simulink model "MotorDriveThermalTestbench"  (R2024b)
settings: Solver=daessc  StartTime=0.0  StopTime=2400  FixedStep=dt  RelTol=1e-3  AbsTol=1e-3
PreLoadFcn:
  | % Simulation parameters
  | MotorDriveThermalTestBenchParams;
model workspace (MAT data in the model file):
  V_frac_bridge = 0.0437
  V_fract_teeth = 0.9563
values from neighbouring files (symbols this model uses):
  CaseParams = struct()    [InverterThermalParams.m]
  HeatsinkParams = struct()    [InverterThermalParams.m]
undefined symbols (not defined in the file or in its folder): electricDrive, H_AH, H_AL, H_BH, H_BL, H_CH, H_CL, PipeParams, vehicleThermal
libraries: fl_lib x171, ee_lib x31, nesl_utility x28, nesl_utility_internal x12, sdl_lib x6, SimscapeFluids_lib x3, autolibshared x1
(part 3 of 4)

== system MotorDriveThermalTestbench/Inverter/AbstractInverter /Inverter Power Module Thermal/HeatSink ==
  Flow Rate Sensor : fl_lib/Thermal Liquid/Sensors/Flow Rate Sensor (TL)  mass_flow_measure=false  volumetric_flow_measure=true  energy_flow_measure=false
      settings: InternalSimscapePortConfiguration="{\"Bottom\":[],\"Left\":[{\"id\":\"A\",\"label\":\"A\",\"type\":\"foundation.thermal_liquid.thermal_liquid\"}],\"Right\":[{\"id\":\"B\",\"label\":\"B\",\"type\":\"foundation.thermal_liquid.thermal_liquid\"},{\"id\":\"V\",\"label\":\"V\",\"type\":\"output\"}],\"Top\":[]}"
  HS Eq Pipe : fl_lib/Thermal Liquid/Elements/Pipe (TL)  length=1.1*HeatsinkParams.ChennelLength m  area=HeatsinkParams.EqPipeDia^2*pi/4 m^2  Dh=HeatsinkParams.EqPipeDia m  length_add=HeatsinkParams.EqLengthRough m  roughness=HeatsinkParams.EqPipeRoughness m  Re_lam=2000  Re_tur=4000  shape_factor=64  Nu_lam=3000  dynamic_compressibility=simscape.enum.onoff.off  inertia=simscape.enum.onoff.off  p0=0.101325 MPa  T0=Tamb degC  mdot0=0 kg/s
  Heatsink : ee_lib/Passive/Thermal/Heatsink  parameterization=ee.enum.passive.thermal.heatsinkParam.rectangularFin  convection=ee.enum.passive.thermal.heatsinkConvection.specifyFlowSpeed  T_vec_Q=[10, 30, 50, 70, 90] K  v_vec_Q=[0, 1, 2, 3] m/s  Q_TLU1=[6.1, 23.6, 44.5, 67.5, 92.3] W  Q_TLU2=[6.1, 18.8, 22.8, 25.7; 23.6, 61.1, 73, 81.5; 44.5, 106.4, 125.9, 140.1; 67.5, 153.5, 180.7, 200.3; 92.3, 202.1, 236.9, 262] W  T_vec_h=[10, 30, 50, 70, 90] K  v_vec_h=[0, 1, 2, 3] m/s  h_TLU1=[5.4, 7.02, 7.98, 8.68, 9.26] W/(K*m^2)  h_TLU2=[5.4, 17.86, 22.17, 25.41; 7.02, 19.49, 23.8, 27.03; 7.97, 20.44, 24.75, 27.99; 8.68, 21.15, 25.46, 28.69; 9.26, 21.73, 26.04, 29.27] W/(K*m^2)  h_vec=[5, 10, 15, 20, 25, 30] W/(K*m^2)  eff_TLU=[96.97, 94.16, 91.53, 89.08, 86.78, 84.62]  height=electricDrive.HeatsinkParams.Height m  thick=electricDrive.HeatsinkParams.Thick m  depth=electricDrive.HeatsinkParams.Depth m  gap=electricDrive.HeatsinkParams.Gap m  num_fins=electricDrive.HeatsinkParams.NumFins  k_fin=386 W/(K*m)  A_total=0.1171 m^2  nu=2.62e-6 m^2/s  alpha=6.55e-8 m^2/s  k_fluid=0.55 W/(K*m)  beta=5.82e-4 1/K  mass=electricDrive.HeatsinkParams.Mass kg  sp_heat=437 J/(K*kg)  T_hs_specify=on  T_hs_priority=High  T_hs=electricDrive.PMparams.TinitCase K  T_hs_nominal_specify=off  T_hs_nominal_value=1  T_hs_nominal_unit=K  Q_A_specify=off  Q_A_priority=None  Q_A=0 W  Q_A_nominal_specify=on  Q_A_nominal_value=1  Q_A_nominal_unit=W  Q_C_specify=off  Q_C_priority=None  Q_C=0 W  Q_C_nominal_specify=on  Q_C_nominal_value=1  Q_C_nominal_unit=W
      settings: InternalSimscapePortConfiguration="{\"Bottom\":[{\"id\":\"C\",\"label\":\"C\",\"type\":\"foundation.thermal.thermal\"}],\"Left\":[{\"id\":\"v\",\"label\":\"v\",\"type\":\"input\"}],\"Right\":[],\"Top\":[{\"id\":\"A\",\"label\":\"A\",\"type\":\"foundation.thermal.thermal\"}]}"
  PS Constant1 : fl_lib/Physical Signals/Sources/PS Constant  constant=PipeParams.Diameter^2*pi/4 m^2
  PS Divide : fl_lib/Physical Signals/Functions/PS Divide
  PS-Simulink Converter : nesl_utility/PS-Simulink Converter  PhysicalDomain=network_engine_domain  SubClassName=ps_output  LeftPortType=input  RightPortType=output  PseudoPeriodic=off  Frequencies=[]  VectorFormat=inherit  Unit=inherit  AffineConversion=off
  Pressure & Temperature Sensor (TL) : fl_lib/Thermal Liquid/Sensors/Pressure & Temperature Sensor (TL)  reference=foundation.enum.MeasurementReference.difference  pressure=true  pressure_spec=foundation.enum.PressureMeasementSpec.Absolute  temperature=true
      settings: InternalSimscapePortConfiguration="{\"Bottom\":[{\"id\":\"T\",\"label\":\"T\",\"type\":\"output\"}],\"Left\":[{\"id\":\"A\",\"label\":\"A\",\"type\":\"foundation.thermal_liquid.thermal_liquid\"}],\"Right\":[{\"id\":\"B\",\"label\":\"B\",\"type\":\"foundation.thermal_liquid.thermal_liquid\"},{\"id\":\"P\",\"label\":\"P\",\"type\":\"output\"}],\"Top\":[]}"
  Scope : Scope
  Hinv : PMIOPort  Side=Left
  coolantIn : PMIOPort  Port=2  Side=Left
  coolantOut : PMIOPort  Port=3  Side=Right
  wires:
  PS-Simulink Converter/1 -> Scope/1
  connections:
  PS Divide/RConn1 -- Heatsink/LConn1
  HS Eq Pipe/LConn1 -- Pressure & Temperature Sensor (TL)/RConn1 -- coolantOut/RConn1
  HS Eq Pipe/RConn1 -- Pressure & Temperature Sensor (TL)/LConn1 -- Flow Rate Sensor/RConn1
  coolantIn/RConn1 -- Flow Rate Sensor/LConn1
  PS Constant1/RConn1 -- PS Divide/LConn2
  Flow Rate Sensor/RConn2 -- PS Divide/LConn1
  HS Eq Pipe/LConn2 -- Heatsink/LConn2
  Hinv/RConn1 -- Heatsink/RConn1
  PS-Simulink Converter/LConn1 -- Pressure & Temperature Sensor (TL)/RConn2

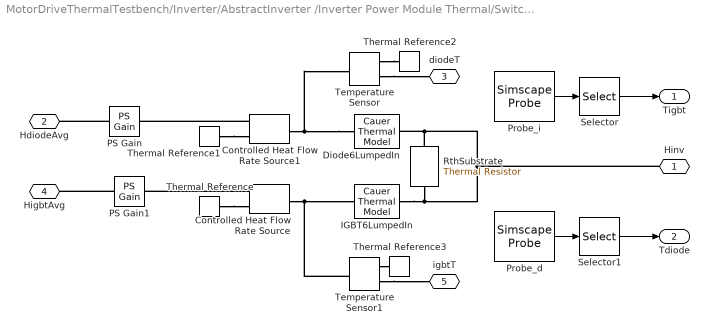
== system MotorDriveThermalTestbench/Inverter/AbstractInverter /Inverter Power Module Thermal/Switches(Averaged IGBT Diode) ==
  Controlled Heat Flow Rate Source : fl_lib/Thermal/Thermal Sources/Controlled Heat Flow Rate Source
  Controlled Heat Flow Rate Source1 : fl_lib/Thermal/Thermal Sources/Controlled Heat Flow Rate Source
  Diode6LumpedIn : ee_lib/Passive/Thermal/Cauer Thermal Model  parameterize_foster=true  resistance_data=1e-3 * [2.6468, 3.8701, 1.2007, .8824] K/W  tau_data=[.0086, .054, .3624, 1.651] s  resistance_data_foster=electricDrive.PMparams.RthDiode K/W  tau_data_foster=electricDrive.PMparams.tauthDiode s  Tvec_specify=on  Tvec_priority=High  Tvec=electricDrive.PMparams.TinitDiode deltaK  Tvec_nominal_specify=off  Tvec_nominal_value=1  Tvec_nominal_unit=K  Q_A_specify=off  Q_A_priority=None  Q_A=0 W  Q_A_nominal_specify=off  Q_A_nominal_value=1  Q_A_nominal_unit=W  Q_B_specify=off  Q_B_priority=None  Q_B=0 W  Q_B_nominal_specify=off  Q_B_nominal_value=1  Q_B_nominal_unit=W
      settings: InternalSimscapePortConfiguration="{\"Bottom\":[],\"Left\":[{\"id\":\"A\",\"label\":\"A\",\"type\":\"foundation.thermal.thermal\"}],\"Right\":[{\"id\":\"B\",\"label\":\"B\",\"type\":\"foundation.thermal.thermal\"}],\"Top\":[]}"
  IGBT6LumpedIn : ee_lib/Passive/Thermal/Cauer Thermal Model  parameterize_foster=true  resistance_data=1e-3 * [2.6468, 3.8701, 1.2007, .8824] K/W  tau_data=[.0086, .054, .3624, 1.651] s  resistance_data_foster=electricDrive.PMparams.RthIGBT K/W  tau_data_foster=electricDrive.PMparams.tauthIGBT s  Tvec_specify=on  Tvec_priority=High  Tvec=electricDrive.PMparams.TinitIGBT deltaK  Tvec_nominal_specify=off  Tvec_nominal_value=1  Tvec_nominal_unit=K  Q_A_specify=off  Q_A_priority=None  Q_A=0 W  Q_A_nominal_specify=off  Q_A_nominal_value=1  Q_A_nominal_unit=W  Q_B_specify=off  Q_B_priority=None  Q_B=0 W  Q_B_nominal_specify=off  Q_B_nominal_value=1  Q_B_nominal_unit=W
      settings: InternalSimscapePortConfiguration="{\"Bottom\":[],\"Left\":[{\"id\":\"A\",\"label\":\"A\",\"type\":\"foundation.thermal.thermal\"}],\"Right\":[{\"id\":\"B\",\"label\":\"B\",\"type\":\"foundation.thermal.thermal\"}],\"Top\":[]}"
  PS Gain : fl_lib/Physical Signals/Functions/PS Gain  gain=6 J/s
  PS Gain1 : fl_lib/Physical Signals/Functions/PS Gain  gain=6 J/s
  Probe_d : SimscapeProbe  BoundBlock=3849  Variables={Tvec}
  Probe_i : SimscapeProbe  BoundBlock=3850  Variables={Tvec}
  RthSubstrate : ee_lib/Passive/Thermal/Thermal Resistor  R=1e-2 K/W  T_specify=off  T_priority=None  T=0 K  T_nominal_specify=off  T_nominal_value=1  T_nominal_unit=K  Q_specify=off  Q_priority=None  Q=0 W  Q_nominal_specify=off  Q_nominal_value=1  Q_nominal_unit=W
      settings: InternalSimscapePortConfiguration="{\"Bottom\":[],\"Left\":[{\"id\":\"A\",\"label\":\"A\",\"type\":\"foundation.thermal.thermal\"}],\"Right\":[{\"id\":\"B\",\"label\":\"B\",\"type\":\"foundation.thermal.thermal\"}],\"Top\":[]}"
  Selector : Selector  InputPortWidth=4  IndexOptions=Index vector (dialog)  Indices=[1]  OutputSizes=1
  Selector1 : Selector  InputPortWidth=4  IndexOptions=Index vector (dialog)  Indices=[1]  OutputSizes=1
  Temperature Sensor : fl_lib/Thermal/Thermal Sensors/Temperature Sensor  temperature_measure=foundation.enum.MeasurementReference.difference
  Temperature Sensor1 : fl_lib/Thermal/Thermal Sensors/Temperature Sensor  temperature_measure=foundation.enum.MeasurementReference.difference
  Thermal Reference{,1..3} (4 alike) : fl_lib/Thermal/Thermal Elements/Thermal Reference
  Hinv : PMIOPort  Side=Left
  HdiodeAvg : PMIOPort  Port=2  Side=Right
  diodeT : PMIOPort  Port=3  Side=Right
  HigbtAvg : PMIOPort  Port=4  Side=Right
  igbtT : PMIOPort  Port=5  Side=Right
  Tigbt : Outport
  Tdiode : Outport  Port=2
  wires:
  Probe_d/1 -> Selector1/1
  Probe_i/1 -> Selector/1
  Selector/1 -> Tigbt/1
  Selector1/1 -> Tdiode/1
  connections:
  Thermal Reference/LConn1 -- Controlled Heat Flow Rate Source/RConn2
  Diode6LumpedIn/LConn1 -- Temperature Sensor/LConn1 -- Controlled Heat Flow Rate Source1/LConn1
  Controlled Heat Flow Rate Source1/RConn1 -- PS Gain/RConn1
  RthSubstrate/LConn1 -- IGBT6LumpedIn/RConn1 -- Hinv/RConn1 -- RthSubstrate/RConn1 -- Diode6LumpedIn/RConn1
  Thermal Reference1/LConn1 -- Controlled Heat Flow Rate Source1/RConn2
  Controlled Heat Flow Rate Source/RConn1 -- PS Gain1/RConn1
  Temperature Sensor/RConn2 -- diodeT/RConn1
  Temperature Sensor/RConn1 -- Thermal Reference2/LConn1
  Temperature Sensor1/RConn1 -- Thermal Reference3/LConn1
  Temperature Sensor1/RConn2 -- igbtT/RConn1
  Temperature Sensor1/LConn1 -- Controlled Heat Flow Rate Source/LConn1 -- IGBT6LumpedIn/LConn1
  PS Gain/LConn1 -- HdiodeAvg/RConn1
  PS Gain1/LConn1 -- HigbtAvg/RConn1

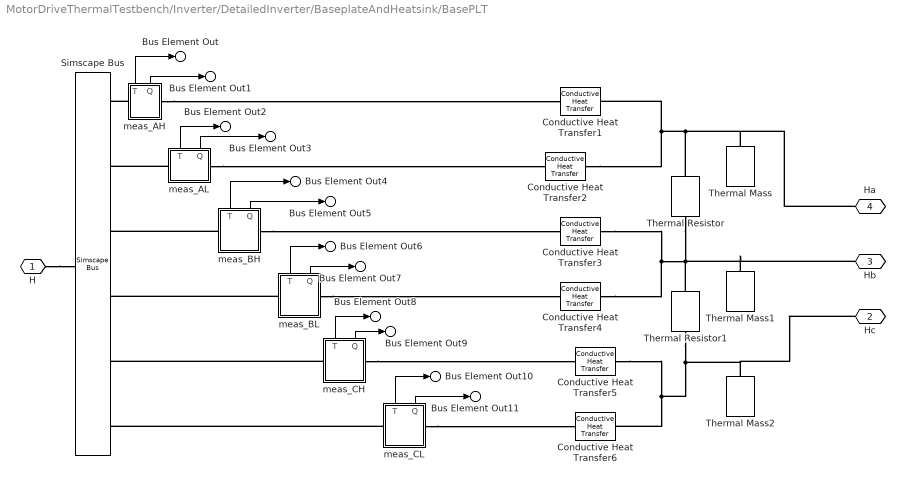
== system MotorDriveThermalTestbench/Inverter/DetailedInverter/BaseplateAndHeatsink/BasePLT ==
  Conductive Heat Transfer{1..6} (6 alike) : fl_lib/Thermal/Thermal Elements/Conductive Heat Transfer  thermal_type=foundation.enum.ConstantVariableTabulated.Constant  wall_geometry=foundation.enum.ConductionWallGeometry.Planar  area=CaseParams.Area m^2  thickness=CaseParams.Thickness m  d_in=0.05 m  d_out=0.1 m  L=1 m  th_cond_min=10 W/(K*m)  th_cond=CaseParams.ThermalConductivity W/(K*m)  th_cond_TLU=[413, 401, 392, 383, 371, 357, 342] W/(K*m)  temp_TLU=[200, 273, 400, 600, 800, 1000, 1200] K  T_specify=off  T_priority=None  T=0 K  T_nominal_specify=off  T_nominal_value=1  T_nominal_unit=K  Q_specify=off  Q_priority=None  Q=0 W  Q_nominal_specify=off  Q_nominal_value=1  Q_nominal_unit=W
  Simscape Bus : SimscapeBus  HierarchyStrings=H_AH;H_AL;H_BH;H_BL;H_CH;H_CL
  Thermal Mass : fl_lib/Thermal/Thermal Elements/Thermal Mass  mass_type=foundation.enum.constant_variable.constant  mass=CaseParams.Mass/3 kg  sp_heat=CaseParams.SpHeat J/(K*kg)  mass_min=1e-6 kg  num_ports=foundation.enum.numPorts2.one  m_specify=off  m_priority=High  m=1 kg  m_nominal_specify=off  m_nominal_value=1  m_nominal_unit=kg  T_specify=on  T_priority=High  T=electricDrive.PMparams.TinitCase K  T_nominal_specify=off  T_nominal_value=1  T_nominal_unit=K  Q_specify=off  Q_priority=None  Q=0 W  Q_nominal_specify=off  Q_nominal_value=1  Q_nominal_unit=W
  Thermal Mass1 : fl_lib/Thermal/Thermal Elements/Thermal Mass  mass_type=foundation.enum.constant_variable.constant  mass=CaseParams.Mass/3 kg  sp_heat=CaseParams.SpHeat J/(K*kg)  mass_min=1e-6 kg  num_ports=foundation.enum.numPorts2.one  m_specify=off  m_priority=High  m=1 kg  m_nominal_specify=off  m_nominal_value=1  m_nominal_unit=kg  T_specify=on  T_priority=High  T=electricDrive.PMparams.TinitCase K  T_nominal_specify=off  T_nominal_value=1  T_nominal_unit=K  Q_specify=off  Q_priority=None  Q=0 W  Q_nominal_specify=off  Q_nominal_value=1  Q_nominal_unit=W
  Thermal Mass2 : fl_lib/Thermal/Thermal Elements/Thermal Mass  mass_type=foundation.enum.constant_variable.constant  mass=CaseParams.Mass/3 kg  sp_heat=CaseParams.SpHeat J/(K*kg)  mass_min=1e-6 kg  num_ports=foundation.enum.numPorts2.one  m_specify=off  m_priority=High  m=1 kg  m_nominal_specify=off  m_nominal_value=1  m_nominal_unit=kg  T_specify=on  T_priority=High  T=electricDrive.PMparams.TinitCase K  T_nominal_specify=off  T_nominal_value=1  T_nominal_unit=K  Q_specify=off  Q_priority=None  Q=0 W  Q_nominal_specify=off  Q_nominal_value=1  Q_nominal_unit=W
  Thermal Resistor : ee_lib/Passive/Thermal/Thermal Resistor  R=1e-1 K/W  T_specify=off  T_priority=None  T=0 K  T_nominal_specify=off  T_nominal_value=1  T_nominal_unit=K  Q_specify=off  Q_priority=None  Q=0 W  Q_nominal_specify=off  Q_nominal_value=1  Q_nominal_unit=W
      settings: InternalSimscapePortConfiguration="{\"Bottom\":[],\"Left\":[{\"id\":\"A\",\"label\":\"A\",\"type\":\"foundation.thermal.thermal\"}],\"Right\":[{\"id\":\"B\",\"label\":\"B\",\"type\":\"foundation.thermal.thermal\"}],\"Top\":[]}"
  Thermal Resistor1 : ee_lib/Passive/Thermal/Thermal Resistor  R=1e-1 K/W  T_specify=off  T_priority=None  T=0 K  T_nominal_specify=off  T_nominal_value=1  T_nominal_unit=K  Q_specify=off  Q_priority=None  Q=0 W  Q_nominal_specify=off  Q_nominal_value=1  Q_nominal_unit=W
      settings: InternalSimscapePortConfiguration="{\"Bottom\":[],\"Left\":[{\"id\":\"A\",\"label\":\"A\",\"type\":\"foundation.thermal.thermal\"}],\"Right\":[{\"id\":\"B\",\"label\":\"B\",\"type\":\"foundation.thermal.thermal\"}],\"Top\":[]}"
  meas_AH : Subsystem
      settings: PortSchema="{\"entries\":[{\"content\":{\"sides\":[{\"content\":{\"connectorIds\":[\"LConn1\"]},\"type\":\"ConnectorPlacement.EquallySpacedRectSide\",\"uuid\":\"1fc63631-1283-41fa-989f-998ad8911336\"},{\"content\":{\"connectorIds\":[\"RConn1\"],\"side\":\"RIGHT\"},\"type\":\"ConnectorPlacement.EquallySpacedRectSide\",\"uuid\":\"60331112-9c9a-4116-97c9-fe3ae6fff227\"},{\"content\":{\"connectorIds\":[\"Out1\",\"Out2\"],\"side\":\"TOP\"},\"type\":\"ConnectorPlacement.EquallySpacedRectSide\",\"uuid\":\"96faf64b-4185-4f1f-9fc5-9c6afe90db96\"}]},\"type\":\"ConnectorPlacement.EquallySpacedConnector\",\"uuid\":\"7d6ee35a-d18e-4643-9192-adf0d71fa59d\"}],\"packageUris\":[\"http://schema.mathworks.com/mf0/Connector/R2020b\"],\"version\":\"1.0\"}"
  meas_AL : Subsystem
      settings: PortSchema="{\"entries\":[{\"content\":{\"sides\":[{\"content\":{\"connectorIds\":[\"LConn1\"]},\"type\":\"ConnectorPlacement.EquallySpacedRectSide\",\"uuid\":\"1fc63631-1283-41fa-989f-998ad8911336\"},{\"content\":{\"connectorIds\":[\"RConn1\"],\"side\":\"RIGHT\"},\"type\":\"ConnectorPlacement.EquallySpacedRectSide\",\"uuid\":\"60331112-9c9a-4116-97c9-fe3ae6fff227\"},{\"content\":{\"connectorIds\":[\"Out1\",\"Out2\"],\"side\":\"TOP\"},\"type\":\"ConnectorPlacement.EquallySpacedRectSide\",\"uuid\":\"96faf64b-4185-4f1f-9fc5-9c6afe90db96\"}]},\"type\":\"ConnectorPlacement.EquallySpacedConnector\",\"uuid\":\"7d6ee35a-d18e-4643-9192-adf0d71fa59d\"}],\"packageUris\":[\"http://schema.mathworks.com/mf0/Connector/R2020b\"],\"version\":\"1.0\"}"
  meas_BH : Subsystem
      settings: PortSchema="{\"entries\":[{\"content\":{\"sides\":[{\"content\":{\"connectorIds\":[\"LConn1\"]},\"type\":\"ConnectorPlacement.EquallySpacedRectSide\",\"uuid\":\"1fc63631-1283-41fa-989f-998ad8911336\"},{\"content\":{\"connectorIds\":[\"RConn1\"],\"side\":\"RIGHT\"},\"type\":\"ConnectorPlacement.EquallySpacedRectSide\",\"uuid\":\"60331112-9c9a-4116-97c9-fe3ae6fff227\"},{\"content\":{\"connectorIds\":[\"Out1\",\"Out2\"],\"side\":\"TOP\"},\"type\":\"ConnectorPlacement.EquallySpacedRectSide\",\"uuid\":\"96faf64b-4185-4f1f-9fc5-9c6afe90db96\"}]},\"type\":\"ConnectorPlacement.EquallySpacedConnector\",\"uuid\":\"7d6ee35a-d18e-4643-9192-adf0d71fa59d\"}],\"packageUris\":[\"http://schema.mathworks.com/mf0/Connector/R2020b\"],\"version\":\"1.0\"}"
  meas_BL : Subsystem
      settings: PortSchema="{\"entries\":[{\"content\":{\"sides\":[{\"content\":{\"connectorIds\":[\"LConn1\"]},\"type\":\"ConnectorPlacement.EquallySpacedRectSide\",\"uuid\":\"1fc63631-1283-41fa-989f-998ad8911336\"},{\"content\":{\"connectorIds\":[\"RConn1\"],\"side\":\"RIGHT\"},\"type\":\"ConnectorPlacement.EquallySpacedRectSide\",\"uuid\":\"60331112-9c9a-4116-97c9-fe3ae6fff227\"},{\"content\":{\"connectorIds\":[\"Out1\",\"Out2\"],\"side\":\"TOP\"},\"type\":\"ConnectorPlacement.EquallySpacedRectSide\",\"uuid\":\"96faf64b-4185-4f1f-9fc5-9c6afe90db96\"}]},\"type\":\"ConnectorPlacement.EquallySpacedConnector\",\"uuid\":\"7d6ee35a-d18e-4643-9192-adf0d71fa59d\"}],\"packageUris\":[\"http://schema.mathworks.com/mf0/Connector/R2020b\"],\"version\":\"1.0\"}"
  meas_CH : Subsystem
      settings: PortSchema="{\"entries\":[{\"content\":{\"sides\":[{\"content\":{\"connectorIds\":[\"LConn1\"]},\"type\":\"ConnectorPlacement.EquallySpacedRectSide\",\"uuid\":\"1fc63631-1283-41fa-989f-998ad8911336\"},{\"content\":{\"connectorIds\":[\"RConn1\"],\"side\":\"RIGHT\"},\"type\":\"ConnectorPlacement.EquallySpacedRectSide\",\"uuid\":\"60331112-9c9a-4116-97c9-fe3ae6fff227\"},{\"content\":{\"connectorIds\":[\"Out1\",\"Out2\"],\"side\":\"TOP\"},\"type\":\"ConnectorPlacement.EquallySpacedRectSide\",\"uuid\":\"96faf64b-4185-4f1f-9fc5-9c6afe90db96\"}]},\"type\":\"ConnectorPlacement.EquallySpacedConnector\",\"uuid\":\"7d6ee35a-d18e-4643-9192-adf0d71fa59d\"}],\"packageUris\":[\"http://schema.mathworks.com/mf0/Connector/R2020b\"],\"version\":\"1.0\"}"
  meas_CL : Subsystem
      settings: PortSchema="{\"entries\":[{\"content\":{\"sides\":[{\"content\":{\"connectorIds\":[\"LConn1\"]},\"type\":\"ConnectorPlacement.EquallySpacedRectSide\",\"uuid\":\"1fc63631-1283-41fa-989f-998ad8911336\"},{\"content\":{\"connectorIds\":[\"RConn1\"],\"side\":\"RIGHT\"},\"type\":\"ConnectorPlacement.EquallySpacedRectSide\",\"uuid\":\"60331112-9c9a-4116-97c9-fe3ae6fff227\"},{\"content\":{\"connectorIds\":[\"Out1\",\"Out2\"],\"side\":\"TOP\"},\"type\":\"ConnectorPlacement.EquallySpacedRectSide\",\"uuid\":\"96faf64b-4185-4f1f-9fc5-9c6afe90db96\"}]},\"type\":\"ConnectorPlacement.EquallySpacedConnector\",\"uuid\":\"7d6ee35a-d18e-4643-9192-adf0d71fa59d\"}],\"packageUris\":[\"http://schema.mathworks.com/mf0/Connector/R2020b\"],\"version\":\"1.0\"}"
  H : PMIOPort  Tag=PMCPort  Side=Left
  Hc : PMIOPort  Port=2  Side=Right
  Hb : PMIOPort  Port=3  Side=Right
  Ha : PMIOPort  Port=4  Side=Right
  Bus Element Out : Outport  PortName=Tmeas  Element=T_AH
  Bus Element Out1 : Outport  PortName=Tmeas  Element=Q_AH
  Bus Element Out2 : Outport  PortName=Tmeas  Element=T_AL
  Bus Element Out3 : Outport  PortName=Tmeas  Element=Q_AL
  Bus Element Out4 : Outport  PortName=Tmeas  Element=T_BH
  Bus Element Out5 : Outport  PortName=Tmeas  Element=Q_BH
  Bus Element Out6 : Outport  PortName=Tmeas  Element=T_BL
  Bus Element Out7 : Outport  PortName=Tmeas  Element=Q_BL
  Bus Element Out8 : Outport  PortName=Tmeas  Element=T_CH
  Bus Element Out9 : Outport  PortName=Tmeas  Element=Q_CH
  Bus Element Out10 : Outport  PortName=Tmeas  Element=T_CL
  Bus Element Out11 : Outport  PortName=Tmeas  Element=Q_CL
  wires:
  meas_AH/1(T) -> Bus Element Out/1
  meas_AH/2(Q) -> Bus Element Out1/1
  meas_AL/1(T) -> Bus Element Out2/1
  meas_AL/2(Q) -> Bus Element Out3/1
  meas_BH/1(T) -> Bus Element Out4/1
  meas_BH/2(Q) -> Bus Element Out5/1
  meas_BL/2(Q) -> Bus Element Out7/1
  meas_BL/1(T) -> Bus Element Out6/1
  meas_CH/2(Q) -> Bus Element Out9/1
  meas_CH/1(T) -> Bus Element Out8/1
  meas_CL/2(Q) -> Bus Element Out11/1
  meas_CL/1(T) -> Bus Element Out10/1
  connections:
  H/RConn1 -- Simscape Bus/RConn1
  Conductive Heat Transfer2/RConn1 -- Thermal Mass/LConn1 -- Ha/RConn1 -- Thermal Resistor/LConn1 -- Conductive Heat Transfer1/RConn1
  meas_AH/RConn1 -- Conductive Heat Transfer1/LConn1
  meas_AH/LConn1 -- Simscape Bus/LConn1
  meas_AL/LConn1 -- Simscape Bus/LConn2
  meas_AL/RConn1 -- Conductive Heat Transfer2/LConn1
  meas_BH/LConn1 -- Simscape Bus/LConn3
  meas_BH/RConn1 -- Conductive Heat Transfer3/LConn1
  meas_BL/RConn1 -- Conductive Heat Transfer4/LConn1
  meas_BL/LConn1 -- Simscape Bus/LConn4
  meas_CH/LConn1 -- Simscape Bus/LConn5
  meas_CH/RConn1 -- Conductive Heat Transfer5/LConn1
  meas_CL/LConn1 -- Simscape Bus/LConn6
  meas_CL/RConn1 -- Conductive Heat Transfer6/LConn1
  Conductive Heat Transfer3/RConn1 -- Conductive Heat Transfer4/RConn1 -- Thermal Resistor/RConn1 -- Thermal Mass1/LConn1 -- Hb/RConn1 -- Thermal Resistor1/LConn1
  Conductive Heat Transfer5/RConn1 -- Thermal Resistor1/RConn1 -- Hc/RConn1 -- Thermal Mass2/LConn1 -- Conductive Heat Transfer6/RConn1

== system MotorDriveThermalTestbench/Inverter/DetailedInverter/BaseplateAndHeatsink/HeatSink ==
  Flow Rate Sensor : fl_lib/Thermal Liquid/Sensors/Flow Rate Sensor (TL)  mass_flow_measure=false  volumetric_flow_measure=true  energy_flow_measure=false
      settings: InternalSimscapePortConfiguration="{\"Bottom\":[],\"Left\":[{\"id\":\"A\",\"label\":\"A\",\"type\":\"foundation.thermal_liquid.thermal_liquid\"}],\"Right\":[{\"id\":\"B\",\"label\":\"B\",\"type\":\"foundation.thermal_liquid.thermal_liquid\"},{\"id\":\"V\",\"label\":\"V\",\"type\":\"output\"}],\"Top\":[]}"
  HeatConduction : Subsystem
  HeatConvection : Subsystem
  PS Divide : fl_lib/Physical Signals/Functions/PS Divide
  PipeArea : fl_lib/Physical Signals/Sources/PS Constant  constant=PipeParams.Diameter^2*pi/4 m^2
  I : PMIOPort  Side=Left
  " Ha" : PMIOPort  Port=2  Side=Left
  Hb : PMIOPort  Port=3  Side=Left
  Hc : PMIOPort  Port=4  Side=Left
  O : PMIOPort  Port=5  Side=Right
  connections:
  HeatConduction/RConn3 -- HeatConvection/LConn4
  HeatConduction/RConn2 -- HeatConvection/LConn3
  Hc/RConn1 -- HeatConduction/LConn4
  Hb/RConn1 -- HeatConduction/LConn3
  HeatConduction/RConn1 -- HeatConvection/LConn2
  O/RConn1 -- HeatConvection/RConn1
  " Ha"/RConn1 -- HeatConduction/LConn2
  PS Divide/RConn1 -- HeatConduction/LConn1
  I/RConn1 -- Flow Rate Sensor/LConn1
  PipeArea/RConn1 -- PS Divide/LConn2
  Flow Rate Sensor/RConn2 -- PS Divide/LConn1
  Flow Rate Sensor/RConn1 -- HeatConvection/LConn1

== system MotorDriveThermalTestbench/Inverter/DetailedInverter/PowerLoss/DiodeLoss ==
  mtq : Inport
  mspd : Inport  Port=2
  temp : Inport  Port=3
  3PhaseDiodeLoss : Subsystem
  DiodeLossTbl : Subsystem
  DutyCycle : Subsystem
  LossDutyCycle : Constant  Value=0.5
  VariablePulse : Subsystem
  Hloss : Outport
  wires:
  3PhaseDiodeLoss/1(Out1) -> Hloss/1
  DutyCycle/4(timeperiod) -> VariablePulse/2(timeperiod)
  DiodeLossTbl/1(Ha) -> 3PhaseDiodeLoss/5(Ha)
  mtq/1 -> DiodeLossTbl/2(mtq)
  temp/1 -> DiodeLossTbl/3(temp)
  DiodeLossTbl/2(Hb) -> 3PhaseDiodeLoss/6(Hb)
  DiodeLossTbl/3(Hc) -> 3PhaseDiodeLoss/7(Hc)
  DutyCycle/5(MotOmega) -> DiodeLossTbl/1(momega)
  LossDutyCycle/1 -> VariablePulse/1(ds)
  DutyCycle/3(d3) -> 3PhaseDiodeLoss/3(d3)
  DutyCycle/2(d2) -> 3PhaseDiodeLoss/2(d2)
  mspd/1 -> DutyCycle/1(motRPM)
  VariablePulse/1(pulse) -> 3PhaseDiodeLoss/4(pls)
  DutyCycle/1(d1) -> 3PhaseDiodeLoss/1(d1)

== system MotorDriveThermalTestbench/Inverter/DetailedInverter/PowerLoss/IGBTloss ==
  mspd : Inport
  mtq : Inport  Port=2
  temp : Inport  Port=3
  3PhaseIGBTLoss : Subsystem
  DutyCycle : Subsystem
  IGBTLossTbl : Subsystem
  LossDutyCycle : Constant  Value=0.5
  VariablePulse : Subsystem
  loss : Outport
  wires:
  mspd/1 -> DutyCycle/1(motRPM)
  VariablePulse/1(pulse) -> 3PhaseIGBTLoss/4(pls)
  DutyCycle/4(timeperiod) -> VariablePulse/2(timeperiod)
  LossDutyCycle/1 -> VariablePulse/1(ds)
  IGBTLossTbl/3(Hc) -> 3PhaseIGBTLoss/7(Hc)
  IGBTLossTbl/2(Hb) -> 3PhaseIGBTLoss/6(Hb)
  temp/1 -> IGBTLossTbl/3(temp)
  DutyCycle/5(MotOmega) -> IGBTLossTbl/1(momega)
  IGBTLossTbl/1(Ha) -> 3PhaseIGBTLoss/5(Ha)
  3PhaseIGBTLoss/1(Out1) -> loss/1
  mtq/1 -> IGBTLossTbl/2(mtq)
  DutyCycle/2(d2) -> 3PhaseIGBTLoss/2(d2)
  DutyCycle/3(d3) -> 3PhaseIGBTLoss/3(d3)
  DutyCycle/1(d1) -> 3PhaseIGBTLoss/1(d1)

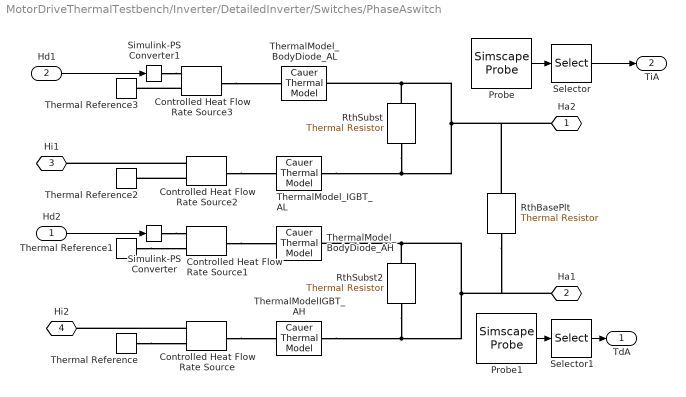
== system MotorDriveThermalTestbench/Inverter/DetailedInverter/Switches/PhaseAswitch ==
  Hd2 : Inport
  Hd1 : Inport  Port=2
  Controlled Heat Flow Rate Source{,1..3} (4 alike) : fl_lib/Thermal/Thermal Sources/Controlled Heat Flow Rate Source
  Probe : SimscapeProbe  BoundBlock=3669  Variables={Tvec}
  Probe1 : SimscapeProbe  BoundBlock=3662  Variables={Tvec}
  RthBasePlt : ee_lib/Passive/Thermal/Thermal Resistor  R=1.04 K/W  T_specify=off  T_priority=None  T=0 K  T_nominal_specify=off  T_nominal_value=1  T_nominal_unit=K  Q_specify=off  Q_priority=None  Q=0 W  Q_nominal_specify=off  Q_nominal_value=1  Q_nominal_unit=W
      settings: InternalSimscapePortConfiguration="{\"Bottom\":[],\"Left\":[{\"id\":\"A\",\"label\":\"A\",\"type\":\"foundation.thermal.thermal\"}],\"Right\":[{\"id\":\"B\",\"label\":\"B\",\"type\":\"foundation.thermal.thermal\"}],\"Top\":[]}"
  RthSubst : ee_lib/Passive/Thermal/Thermal Resistor  R=0.26 K/W  T_specify=off  T_priority=None  T=0 K  T_nominal_specify=off  T_nominal_value=1  T_nominal_unit=K  Q_specify=off  Q_priority=None  Q=0 W  Q_nominal_specify=off  Q_nominal_value=1  Q_nominal_unit=W
      settings: InternalSimscapePortConfiguration="{\"Bottom\":[],\"Left\":[{\"id\":\"A\",\"label\":\"A\",\"type\":\"foundation.thermal.thermal\"}],\"Right\":[{\"id\":\"B\",\"label\":\"B\",\"type\":\"foundation.thermal.thermal\"}],\"Top\":[]}"
  RthSubst2 : ee_lib/Passive/Thermal/Thermal Resistor  R=0.26 K/W  T_specify=off  T_priority=None  T=0 K  T_nominal_specify=off  T_nominal_value=1  T_nominal_unit=K  Q_specify=off  Q_priority=None  Q=0 W  Q_nominal_specify=off  Q_nominal_value=1  Q_nominal_unit=W
      settings: InternalSimscapePortConfiguration="{\"Bottom\":[],\"Left\":[{\"id\":\"A\",\"label\":\"A\",\"type\":\"foundation.thermal.thermal\"}],\"Right\":[{\"id\":\"B\",\"label\":\"B\",\"type\":\"foundation.thermal.thermal\"}],\"Top\":[]}"
  Selector : Selector  InputPortWidth=4  IndexOptions=Index vector (dialog)  Indices=[1]  OutputSizes=1
  Selector1 : Selector  InputPortWidth=4  IndexOptions=Index vector (dialog)  Indices=[1]  OutputSizes=1
  Simulink-PS Converter : nesl_utility/Simulink-PS Converter  PhysicalDomain=network_engine_domain  SubClassName=ps_input  LeftPortType=input  RightPortType=output  PseudoPeriodic=off  Frequencies=[]  NoiseDistribution=none  NoiseParameters=[]  Unit=J/s  AffineConversion=off  FilteringAndDerivatives=provide  SimscapeFilterOrder=1  InputFilterTimeConstant=0.001  UdotUserProvided=0
  Simulink-PS Converter1 : nesl_utility/Simulink-PS Converter  PhysicalDomain=network_engine_domain  SubClassName=ps_input  LeftPortType=input  RightPortType=output  PseudoPeriodic=off  Frequencies=[]  NoiseDistribution=none  NoiseParameters=[]  Unit=J/s  AffineConversion=off  FilteringAndDerivatives=provide  SimscapeFilterOrder=1  InputFilterTimeConstant=0.001  UdotUserProvided=0
  Thermal Reference{,1..3} (4 alike) : fl_lib/Thermal/Thermal Elements/Thermal Reference
  ThermalModelIGBT_AH : ee_lib/Passive/Thermal/Cauer Thermal Model  parameterize_foster=true  resistance_data=1e-3 * [2.6468, 3.8701, 1.2007, .8824] K/W  tau_data=[.0086, .054, .3624, 1.651] s  resistance_data_foster=RthIGBT K/W  tau_data_foster=tauthIGBT s  Tvec_specify=on  Tvec_priority=High  Tvec=electricDrive.PMparams.TinitIGBT K  Tvec_nominal_specify=off  Tvec_nominal_value=1  Tvec_nominal_unit=K  Q_A_specify=off  Q_A_priority=None  Q_A=0 W  Q_A_nominal_specify=off  Q_A_nominal_value=1  Q_A_nominal_unit=W  Q_B_specify=off  Q_B_priority=None  Q_B=0 W  Q_B_nominal_specify=off  Q_B_nominal_value=1  Q_B_nominal_unit=W
      settings: InternalSimscapePortConfiguration="{\"Bottom\":[],\"Left\":[{\"id\":\"A\",\"label\":\"A\",\"type\":\"foundation.thermal.thermal\"}],\"Right\":[{\"id\":\"B\",\"label\":\"B\",\"type\":\"foundation.thermal.thermal\"}],\"Top\":[]}"
  ThermalModel_BodyDiode_AH : ee_lib/Passive/Thermal/Cauer Thermal Model  parameterize_foster=true  resistance_data=1e-3 * [2.6468, 3.8701, 1.2007, .8824] K/W  tau_data=[.0086, .054, .3624, 1.651] s  resistance_data_foster=RthDiode K/W  tau_data_foster=tauthDiode s  Tvec_specify=on  Tvec_priority=High  Tvec=electricDrive.PMparams.TinitDiode K  Tvec_nominal_specify=off  Tvec_nominal_value=1  Tvec_nominal_unit=K  Q_A_specify=off  Q_A_priority=None  Q_A=0 W  Q_A_nominal_specify=off  Q_A_nominal_value=1  Q_A_nominal_unit=W  Q_B_specify=off  Q_B_priority=None  Q_B=0 W  Q_B_nominal_specify=off  Q_B_nominal_value=1  Q_B_nominal_unit=W
      settings: InternalSimscapePortConfiguration="{\"Bottom\":[],\"Left\":[{\"id\":\"A\",\"label\":\"A\",\"type\":\"foundation.thermal.thermal\"}],\"Right\":[{\"id\":\"B\",\"label\":\"B\",\"type\":\"foundation.thermal.thermal\"}],\"Top\":[]}"
  ThermalModel_BodyDiode_AL : ee_lib/Passive/Thermal/Cauer Thermal Model  parameterize_foster=true  resistance_data=1e-3 * [2.6468, 3.8701, 1.2007, .8824] K/W  tau_data=[.0086, .054, .3624, 1.651] s  resistance_data_foster=RthDiode K/W  tau_data_foster=tauthDiode s  Tvec_specify=on  Tvec_priority=High  Tvec=electricDrive.PMparams.TinitDiode K  Tvec_nominal_specify=off  Tvec_nominal_value=1  Tvec_nominal_unit=K  Q_A_specify=off  Q_A_priority=None  Q_A=0 W  Q_A_nominal_specify=off  Q_A_nominal_value=1  Q_A_nominal_unit=W  Q_B_specify=off  Q_B_priority=None  Q_B=0 W  Q_B_nominal_specify=off  Q_B_nominal_value=1  Q_B_nominal_unit=W
      settings: InternalSimscapePortConfiguration="{\"Bottom\":[],\"Left\":[{\"id\":\"A\",\"label\":\"A\",\"type\":\"foundation.thermal.thermal\"}],\"Right\":[{\"id\":\"B\",\"label\":\"B\",\"type\":\"foundation.thermal.thermal\"}],\"Top\":[]}"
  ThermalModel_IGBT_AL : ee_lib/Passive/Thermal/Cauer Thermal Model  parameterize_foster=true  resistance_data=1e-3 * [2.6468, 3.8701, 1.2007, .8824] K/W  tau_data=[.0086, .054, .3624, 1.651] s  resistance_data_foster=RthIGBT K/W  tau_data_foster=tauthIGBT s  Tvec_specify=on  Tvec_priority=High  Tvec=electricDrive.PMparams.TinitIGBT K  Tvec_nominal_specify=off  Tvec_nominal_value=1  Tvec_nominal_unit=K  Q_A_specify=off  Q_A_priority=None  Q_A=0 W  Q_A_nominal_specify=off  Q_A_nominal_value=1  Q_A_nominal_unit=W  Q_B_specify=off  Q_B_priority=None  Q_B=0 W  Q_B_nominal_specify=off  Q_B_nominal_value=1  Q_B_nominal_unit=W
      settings: InternalSimscapePortConfiguration="{\"Bottom\":[],\"Left\":[{\"id\":\"A\",\"label\":\"A\",\"type\":\"foundation.thermal.thermal\"}],\"Right\":[{\"id\":\"B\",\"label\":\"B\",\"type\":\"foundation.thermal.thermal\"}],\"Top\":[]}"
  Ha2 : PMIOPort  Side=Left
  Ha1 : PMIOPort  Port=2  Side=Left
  Hi1 : PMIOPort  Port=3  Side=Right
  Hi2 : PMIOPort  Port=4  Side=Right
  TdA : Outport
  TiA : Outport  Port=2
  wires:
  Hd2/1 -> Simulink-PS Converter/1
  Hd1/1 -> Simulink-PS Converter1/1
  Probe/1 -> Selector/1
  Probe1/1 -> Selector1/1
  Selector/1 -> TiA/1
  Selector1/1 -> TdA/1
  connections:
  ThermalModel_IGBT_AL/RConn1 -- RthSubst/LConn1 -- RthBasePlt/RConn1 -- Ha2/RConn1 -- RthSubst/RConn1 -- ThermalModel_BodyDiode_AL/RConn1
  ThermalModelIGBT_AH/RConn1 -- RthSubst2/LConn1 -- RthBasePlt/LConn1 -- Ha1/RConn1 -- RthSubst2/RConn1 -- ThermalModel_BodyDiode_AH/RConn1
  Controlled Heat Flow Rate Source1/LConn1 -- ThermalModel_BodyDiode_AH/LConn1
  Controlled Heat Flow Rate Source/RConn1 -- Hi2/RConn1
  Controlled Heat Flow Rate Source2/LConn1 -- ThermalModel_IGBT_AL/LConn1
  Controlled Heat Flow Rate Source2/RConn2 -- Thermal Reference2/LConn1
  Controlled Heat Flow Rate Source/LConn1 -- ThermalModelIGBT_AH/LConn1
  Controlled Heat Flow Rate Source3/LConn1 -- ThermalModel_BodyDiode_AL/LConn1
  Thermal Reference/LConn1 -- Controlled Heat Flow Rate Source/RConn2
  Controlled Heat Flow Rate Source3/RConn2 -- Thermal Reference3/LConn1
  Simulink-PS Converter/RConn1 -- Controlled Heat Flow Rate Source1/RConn1
  Controlled Heat Flow Rate Source2/RConn1 -- Hi1/RConn1
  Simulink-PS Converter1/RConn1 -- Controlled Heat Flow Rate Source3/RConn1
  Thermal Reference1/LConn1 -- Controlled Heat Flow Rate Source1/RConn2

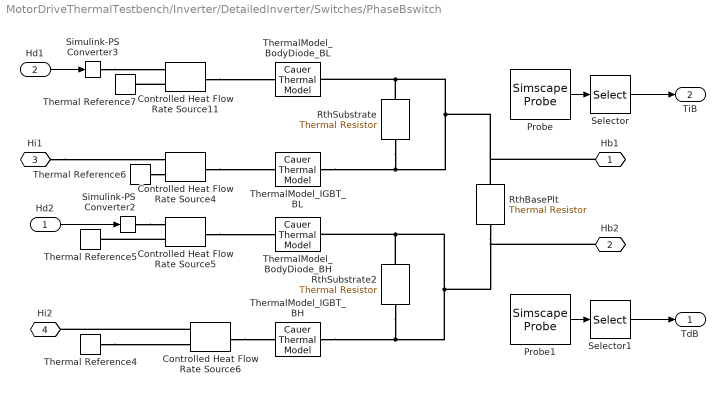
== system MotorDriveThermalTestbench/Inverter/DetailedInverter/Switches/PhaseBswitch ==
  Hd2 : Inport
  Hd1 : Inport  Port=2
  Controlled Heat Flow Rate Source{4..6,11} (4 alike) : fl_lib/Thermal/Thermal Sources/Controlled Heat Flow Rate Source
  Probe : SimscapeProbe  BoundBlock=3671  Variables={Tvec}
  Probe1 : SimscapeProbe  BoundBlock=3664  Variables={Tvec}
  RthBasePlt : ee_lib/Passive/Thermal/Thermal Resistor  R=1.04 K/W  T_specify=off  T_priority=None  T=0 K  T_nominal_specify=off  T_nominal_value=1  T_nominal_unit=K  Q_specify=off  Q_priority=None  Q=0 W  Q_nominal_specify=off  Q_nominal_value=1  Q_nominal_unit=W
      settings: InternalSimscapePortConfiguration="{\"Bottom\":[],\"Left\":[{\"id\":\"A\",\"label\":\"A\",\"type\":\"foundation.thermal.thermal\"}],\"Right\":[{\"id\":\"B\",\"label\":\"B\",\"type\":\"foundation.thermal.thermal\"}],\"Top\":[]}"
  RthSubstrate : ee_lib/Passive/Thermal/Thermal Resistor  R=0.26 K/W  T_specify=off  T_priority=None  T=0 K  T_nominal_specify=off  T_nominal_value=1  T_nominal_unit=K  Q_specify=off  Q_priority=None  Q=0 W  Q_nominal_specify=off  Q_nominal_value=1  Q_nominal_unit=W
      settings: InternalSimscapePortConfiguration="{\"Bottom\":[],\"Left\":[{\"id\":\"A\",\"label\":\"A\",\"type\":\"foundation.thermal.thermal\"}],\"Right\":[{\"id\":\"B\",\"label\":\"B\",\"type\":\"foundation.thermal.thermal\"}],\"Top\":[]}"
  RthSubstrate2 : ee_lib/Passive/Thermal/Thermal Resistor  R=0.26 K/W  T_specify=off  T_priority=None  T=0 K  T_nominal_specify=off  T_nominal_value=1  T_nominal_unit=K  Q_specify=off  Q_priority=None  Q=0 W  Q_nominal_specify=off  Q_nominal_value=1  Q_nominal_unit=W
      settings: InternalSimscapePortConfiguration="{\"Bottom\":[],\"Left\":[{\"id\":\"A\",\"label\":\"A\",\"type\":\"foundation.thermal.thermal\"}],\"Right\":[{\"id\":\"B\",\"label\":\"B\",\"type\":\"foundation.thermal.thermal\"}],\"Top\":[]}"
  Selector : Selector  InputPortWidth=4  IndexOptions=Index vector (dialog)  Indices=[1]  OutputSizes=1
  Selector1 : Selector  InputPortWidth=4  IndexOptions=Index vector (dialog)  Indices=[1]  OutputSizes=1
  Simulink-PS Converter2 : nesl_utility/Simulink-PS Converter  PhysicalDomain=network_engine_domain  SubClassName=ps_input  LeftPortType=input  RightPortType=output  PseudoPeriodic=off  Frequencies=[]  NoiseDistribution=none  NoiseParameters=[]  Unit=J/s  AffineConversion=off  FilteringAndDerivatives=provide  SimscapeFilterOrder=1  InputFilterTimeConstant=0.001  UdotUserProvided=0
  Simulink-PS Converter3 : nesl_utility/Simulink-PS Converter  PhysicalDomain=network_engine_domain  SubClassName=ps_input  LeftPortType=input  RightPortType=output  PseudoPeriodic=off  Frequencies=[]  NoiseDistribution=none  NoiseParameters=[]  Unit=J/s  AffineConversion=off  FilteringAndDerivatives=provide  SimscapeFilterOrder=1  InputFilterTimeConstant=0.001  UdotUserProvided=0
  Thermal Reference{4..7} (4 alike) : fl_lib/Thermal/Thermal Elements/Thermal Reference
  ThermalModel_BodyDiode_BH : ee_lib/Passive/Thermal/Cauer Thermal Model  parameterize_foster=true  resistance_data=1e-3 * [2.6468, 3.8701, 1.2007, .8824] K/W  tau_data=[.0086, .054, .3624, 1.651] s  resistance_data_foster=RthDiode K/W  tau_data_foster=tauthDiode s  Tvec_specify=on  Tvec_priority=High  Tvec=electricDrive.PMparams.TinitDiode K  Tvec_nominal_specify=off  Tvec_nominal_value=1  Tvec_nominal_unit=K  Q_A_specify=off  Q_A_priority=None  Q_A=0 W  Q_A_nominal_specify=off  Q_A_nominal_value=1  Q_A_nominal_unit=W  Q_B_specify=off  Q_B_priority=None  Q_B=0 W  Q_B_nominal_specify=off  Q_B_nominal_value=1  Q_B_nominal_unit=W
      settings: InternalSimscapePortConfiguration="{\"Bottom\":[],\"Left\":[{\"id\":\"A\",\"label\":\"A\",\"type\":\"foundation.thermal.thermal\"}],\"Right\":[{\"id\":\"B\",\"label\":\"B\",\"type\":\"foundation.thermal.thermal\"}],\"Top\":[]}"
  ThermalModel_BodyDiode_BL : ee_lib/Passive/Thermal/Cauer Thermal Model  parameterize_foster=true  resistance_data=1e-3 * [2.6468, 3.8701, 1.2007, .8824] K/W  tau_data=[.0086, .054, .3624, 1.651] s  resistance_data_foster=RthDiode K/W  tau_data_foster=tauthDiode s  Tvec_specify=on  Tvec_priority=High  Tvec=electricDrive.PMparams.TinitDiode K  Tvec_nominal_specify=off  Tvec_nominal_value=1  Tvec_nominal_unit=K  Q_A_specify=off  Q_A_priority=None  Q_A=0 W  Q_A_nominal_specify=off  Q_A_nominal_value=1  Q_A_nominal_unit=W  Q_B_specify=off  Q_B_priority=None  Q_B=0 W  Q_B_nominal_specify=off  Q_B_nominal_value=1  Q_B_nominal_unit=W
      settings: InternalSimscapePortConfiguration="{\"Bottom\":[],\"Left\":[{\"id\":\"A\",\"label\":\"A\",\"type\":\"foundation.thermal.thermal\"}],\"Right\":[{\"id\":\"B\",\"label\":\"B\",\"type\":\"foundation.thermal.thermal\"}],\"Top\":[]}"
  ThermalModel_IGBT_BH : ee_lib/Passive/Thermal/Cauer Thermal Model  parameterize_foster=true  resistance_data=1e-3 * [2.6468, 3.8701, 1.2007, .8824] K/W  tau_data=[.0086, .054, .3624, 1.651] s  resistance_data_foster=RthIGBT K/W  tau_data_foster=tauthIGBT s  Tvec_specify=on  Tvec_priority=High  Tvec=electricDrive.PMparams.TinitIGBT K  Tvec_nominal_specify=off  Tvec_nominal_value=1  Tvec_nominal_unit=K  Q_A_specify=off  Q_A_priority=None  Q_A=0 W  Q_A_nominal_specify=off  Q_A_nominal_value=1  Q_A_nominal_unit=W  Q_B_specify=off  Q_B_priority=None  Q_B=0 W  Q_B_nominal_specify=off  Q_B_nominal_value=1  Q_B_nominal_unit=W
      settings: InternalSimscapePortConfiguration="{\"Bottom\":[],\"Left\":[{\"id\":\"A\",\"label\":\"A\",\"type\":\"foundation.thermal.thermal\"}],\"Right\":[{\"id\":\"B\",\"label\":\"B\",\"type\":\"foundation.thermal.thermal\"}],\"Top\":[]}"
  ThermalModel_IGBT_BL : ee_lib/Passive/Thermal/Cauer Thermal Model  parameterize_foster=true  resistance_data=1e-3 * [2.6468, 3.8701, 1.2007, .8824] K/W  tau_data=[.0086, .054, .3624, 1.651] s  resistance_data_foster=RthIGBT K/W  tau_data_foster=tauthIGBT s  Tvec_specify=on  Tvec_priority=High  Tvec=electricDrive.PMparams.TinitIGBT K  Tvec_nominal_specify=off  Tvec_nominal_value=1  Tvec_nominal_unit=K  Q_A_specify=off  Q_A_priority=None  Q_A=0 W  Q_A_nominal_specify=off  Q_A_nominal_value=1  Q_A_nominal_unit=W  Q_B_specify=off  Q_B_priority=None  Q_B=0 W  Q_B_nominal_specify=off  Q_B_nominal_value=1  Q_B_nominal_unit=W
      settings: InternalSimscapePortConfiguration="{\"Bottom\":[],\"Left\":[{\"id\":\"A\",\"label\":\"A\",\"type\":\"foundation.thermal.thermal\"}],\"Right\":[{\"id\":\"B\",\"label\":\"B\",\"type\":\"foundation.thermal.thermal\"}],\"Top\":[]}"
  Hb1 : PMIOPort  Side=Left
  Hb2 : PMIOPort  Port=2  Side=Left
  Hi1 : PMIOPort  Port=3  Side=Right
  Hi2 : PMIOPort  Port=4  Side=Right
  TdB : Outport
  TiB : Outport  Port=2
  wires:
  Hd1/1 -> Simulink-PS Converter3/1
  Hd2/1 -> Simulink-PS Converter2/1
  Probe/1 -> Selector/1
  Selector/1 -> TiB/1
  Probe1/1 -> Selector1/1
  Selector1/1 -> TdB/1
  connections:
  ThermalModel_IGBT_BH/RConn1 -- RthSubstrate2/LConn1 -- Hb2/RConn1 -- RthBasePlt/LConn1 -- RthSubstrate2/RConn1 -- ThermalModel_BodyDiode_BH/RConn1
  Controlled Heat Flow Rate Source11/LConn1 -- ThermalModel_BodyDiode_BL/LConn1
  ThermalModel_IGBT_BL/RConn1 -- RthSubstrate/LConn1 -- Hb1/RConn1 -- RthBasePlt/RConn1 -- ThermalModel_BodyDiode_BL/RConn1 -- RthSubstrate/RConn1
  Thermal Reference4/LConn1 -- Controlled Heat Flow Rate Source6/RConn2
  Controlled Heat Flow Rate Source5/LConn1 -- ThermalModel_BodyDiode_BH/LConn1
  Controlled Heat Flow Rate Source4/LConn1 -- ThermalModel_IGBT_BL/LConn1
  Controlled Heat Flow Rate Source5/RConn2 -- Thermal Reference5/LConn1
  Thermal Reference6/LConn1 -- Controlled Heat Flow Rate Source4/RConn2
  Simulink-PS Converter3/RConn1 -- Controlled Heat Flow Rate Source11/RConn1
  Controlled Heat Flow Rate Source6/RConn1 -- Hi2/RConn1
  Controlled Heat Flow Rate Source6/LConn1 -- ThermalModel_IGBT_BH/LConn1
  Simulink-PS Converter2/RConn1 -- Controlled Heat Flow Rate Source5/RConn1
  Controlled Heat Flow Rate Source11/RConn2 -- Thermal Reference7/LConn1
  Hi1/RConn1 -- Controlled Heat Flow Rate Source4/RConn1

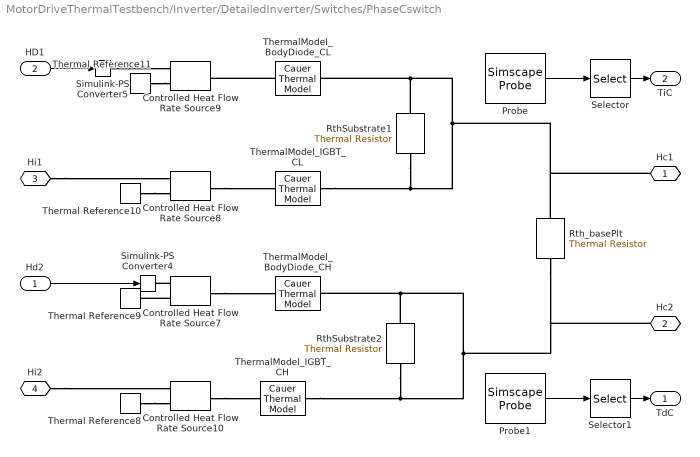
== system MotorDriveThermalTestbench/Inverter/DetailedInverter/Switches/PhaseCswitch ==
  Hd2 : Inport
  HD1 : Inport  Port=2
  Controlled Heat Flow Rate Source{7..10} (4 alike) : fl_lib/Thermal/Thermal Sources/Controlled Heat Flow Rate Source
  Probe : SimscapeProbe  BoundBlock=3673  Variables={Tvec}
  Probe1 : SimscapeProbe  BoundBlock=3666  Variables={Tvec}
  RthSubstrate1 : ee_lib/Passive/Thermal/Thermal Resistor  R=0.26 K/W  T_specify=off  T_priority=None  T=0 K  T_nominal_specify=off  T_nominal_value=1  T_nominal_unit=K  Q_specify=off  Q_priority=None  Q=0 W  Q_nominal_specify=off  Q_nominal_value=1  Q_nominal_unit=W
      settings: InternalSimscapePortConfiguration="{\"Bottom\":[],\"Left\":[{\"id\":\"A\",\"label\":\"A\",\"type\":\"foundation.thermal.thermal\"}],\"Right\":[{\"id\":\"B\",\"label\":\"B\",\"type\":\"foundation.thermal.thermal\"}],\"Top\":[]}"
  RthSubstrate2 : ee_lib/Passive/Thermal/Thermal Resistor  R=0.26 K/W  T_specify=off  T_priority=None  T=0 K  T_nominal_specify=off  T_nominal_value=1  T_nominal_unit=K  Q_specify=off  Q_priority=None  Q=0 W  Q_nominal_specify=off  Q_nominal_value=1  Q_nominal_unit=W
      settings: InternalSimscapePortConfiguration="{\"Bottom\":[],\"Left\":[{\"id\":\"A\",\"label\":\"A\",\"type\":\"foundation.thermal.thermal\"}],\"Right\":[{\"id\":\"B\",\"label\":\"B\",\"type\":\"foundation.thermal.thermal\"}],\"Top\":[]}"
  Rth_basePlt : ee_lib/Passive/Thermal/Thermal Resistor  R=1.04 K/W  T_specify=off  T_priority=None  T=0 K  T_nominal_specify=off  T_nominal_value=1  T_nominal_unit=K  Q_specify=off  Q_priority=None  Q=0 W  Q_nominal_specify=off  Q_nominal_value=1  Q_nominal_unit=W
      settings: InternalSimscapePortConfiguration="{\"Bottom\":[],\"Left\":[{\"id\":\"A\",\"label\":\"A\",\"type\":\"foundation.thermal.thermal\"}],\"Right\":[{\"id\":\"B\",\"label\":\"B\",\"type\":\"foundation.thermal.thermal\"}],\"Top\":[]}"
  Selector : Selector  InputPortWidth=4  IndexOptions=Index vector (dialog)  Indices=[1]  OutputSizes=1
  Selector1 : Selector  InputPortWidth=4  IndexOptions=Index vector (dialog)  Indices=[1]  OutputSizes=1
  Simulink-PS Converter4 : nesl_utility/Simulink-PS Converter  PhysicalDomain=network_engine_domain  SubClassName=ps_input  LeftPortType=input  RightPortType=output  PseudoPeriodic=off  Frequencies=[]  NoiseDistribution=none  NoiseParameters=[]  Unit=J/s  AffineConversion=off  FilteringAndDerivatives=provide  SimscapeFilterOrder=1  InputFilterTimeConstant=0.001  UdotUserProvided=0
  Simulink-PS Converter5 : nesl_utility/Simulink-PS Converter  PhysicalDomain=network_engine_domain  SubClassName=ps_input  LeftPortType=input  RightPortType=output  PseudoPeriodic=off  Frequencies=[]  NoiseDistribution=none  NoiseParameters=[]  Unit=J/s  AffineConversion=off  FilteringAndDerivatives=provide  SimscapeFilterOrder=1  InputFilterTimeConstant=0.001  UdotUserProvided=0
  Thermal Reference{8..11} (4 alike) : fl_lib/Thermal/Thermal Elements/Thermal Reference
  ThermalModel_BodyDiode_CH : ee_lib/Passive/Thermal/Cauer Thermal Model  parameterize_foster=true  resistance_data=1e-3 * [2.6468, 3.8701, 1.2007, .8824] K/W  tau_data=[.0086, .054, .3624, 1.651] s  resistance_data_foster=RthDiode K/W  tau_data_foster=tauthDiode s  Tvec_specify=on  Tvec_priority=High  Tvec=electricDrive.PMparams.TinitDiode K  Tvec_nominal_specify=off  Tvec_nominal_value=1  Tvec_nominal_unit=K  Q_A_specify=off  Q_A_priority=None  Q_A=0 W  Q_A_nominal_specify=off  Q_A_nominal_value=1  Q_A_nominal_unit=W  Q_B_specify=off  Q_B_priority=None  Q_B=0 W  Q_B_nominal_specify=off  Q_B_nominal_value=1  Q_B_nominal_unit=W
      settings: InternalSimscapePortConfiguration="{\"Bottom\":[],\"Left\":[{\"id\":\"A\",\"label\":\"A\",\"type\":\"foundation.thermal.thermal\"}],\"Right\":[{\"id\":\"B\",\"label\":\"B\",\"type\":\"foundation.thermal.thermal\"}],\"Top\":[]}"
  ThermalModel_BodyDiode_CL : ee_lib/Passive/Thermal/Cauer Thermal Model  parameterize_foster=true  resistance_data=1e-3 * [2.6468, 3.8701, 1.2007, .8824] K/W  tau_data=[.0086, .054, .3624, 1.651] s  resistance_data_foster=RthDiode K/W  tau_data_foster=tauthDiode s  Tvec_specify=on  Tvec_priority=High  Tvec=electricDrive.PMparams.TinitDiode K  Tvec_nominal_specify=off  Tvec_nominal_value=1  Tvec_nominal_unit=K  Q_A_specify=off  Q_A_priority=None  Q_A=0 W  Q_A_nominal_specify=off  Q_A_nominal_value=1  Q_A_nominal_unit=W  Q_B_specify=off  Q_B_priority=None  Q_B=0 W  Q_B_nominal_specify=off  Q_B_nominal_value=1  Q_B_nominal_unit=W
      settings: InternalSimscapePortConfiguration="{\"Bottom\":[],\"Left\":[{\"id\":\"A\",\"label\":\"A\",\"type\":\"foundation.thermal.thermal\"}],\"Right\":[{\"id\":\"B\",\"label\":\"B\",\"type\":\"foundation.thermal.thermal\"}],\"Top\":[]}"
  ThermalModel_IGBT_CH : ee_lib/Passive/Thermal/Cauer Thermal Model  parameterize_foster=true  resistance_data=1e-3 * [2.6468, 3.8701, 1.2007, .8824] K/W  tau_data=[.0086, .054, .3624, 1.651] s  resistance_data_foster=RthIGBT K/W  tau_data_foster=tauthIGBT s  Tvec_specify=on  Tvec_priority=High  Tvec=electricDrive.PMparams.TinitIGBT K  Tvec_nominal_specify=off  Tvec_nominal_value=1  Tvec_nominal_unit=K  Q_A_specify=off  Q_A_priority=None  Q_A=0 W  Q_A_nominal_specify=off  Q_A_nominal_value=1  Q_A_nominal_unit=W  Q_B_specify=off  Q_B_priority=None  Q_B=0 W  Q_B_nominal_specify=off  Q_B_nominal_value=1  Q_B_nominal_unit=W
      settings: InternalSimscapePortConfiguration="{\"Bottom\":[],\"Left\":[{\"id\":\"A\",\"label\":\"A\",\"type\":\"foundation.thermal.thermal\"}],\"Right\":[{\"id\":\"B\",\"label\":\"B\",\"type\":\"foundation.thermal.thermal\"}],\"Top\":[]}"
  ThermalModel_IGBT_CL : ee_lib/Passive/Thermal/Cauer Thermal Model  parameterize_foster=true  resistance_data=1e-3 * [2.6468, 3.8701, 1.2007, .8824] K/W  tau_data=[.0086, .054, .3624, 1.651] s  resistance_data_foster=RthIGBT K/W  tau_data_foster=tauthIGBT s  Tvec_specify=on  Tvec_priority=High  Tvec=electricDrive.PMparams.TinitIGBT K  Tvec_nominal_specify=off  Tvec_nominal_value=1  Tvec_nominal_unit=K  Q_A_specify=off  Q_A_priority=None  Q_A=0 W  Q_A_nominal_specify=off  Q_A_nominal_value=1  Q_A_nominal_unit=W  Q_B_specify=off  Q_B_priority=None  Q_B=0 W  Q_B_nominal_specify=off  Q_B_nominal_value=1  Q_B_nominal_unit=W
      settings: InternalSimscapePortConfiguration="{\"Bottom\":[],\"Left\":[{\"id\":\"A\",\"label\":\"A\",\"type\":\"foundation.thermal.thermal\"}],\"Right\":[{\"id\":\"B\",\"label\":\"B\",\"type\":\"foundation.thermal.thermal\"}],\"Top\":[]}"
  "Hc1 " : PMIOPort  Side=Left
  "Hc2 " : PMIOPort  Port=2  Side=Left
  Hi1 : PMIOPort  Port=3  Side=Right
  Hi2 : PMIOPort  Port=4  Side=Right
  " TdC" : Outport
  TiC : Outport  Port=2
  wires:
  Hd2/1 -> Simulink-PS Converter4/1
  HD1/1 -> Simulink-PS Converter5/1
  Probe/1 -> Selector/1
  Selector/1 -> TiC/1
  Probe1/1 -> Selector1/1
  Selector1/1 -> " TdC"/1
  connections:
  Controlled Heat Flow Rate Source8/LConn1 -- ThermalModel_IGBT_CL/LConn1
  Thermal Reference8/LConn1 -- Controlled Heat Flow Rate Source10/RConn2
  ThermalModel_IGBT_CH/RConn1 -- "Hc2 "/RConn1 -- Rth_basePlt/LConn1 -- RthSubstrate2/RConn1 -- ThermalModel_BodyDiode_CH/RConn1 -- RthSubstrate2/LConn1
  ThermalModel_BodyDiode_CL/LConn1 -- Controlled Heat Flow Rate Source9/LConn1
  Thermal Reference11/LConn1 -- Controlled Heat Flow Rate Source9/RConn2
  Hi2/RConn1 -- Controlled Heat Flow Rate Source10/RConn1
  Controlled Heat Flow Rate Source10/LConn1 -- ThermalModel_IGBT_CH/LConn1
  Thermal Reference10/LConn1 -- Controlled Heat Flow Rate Source8/RConn2
  ThermalModel_IGBT_CL/RConn1 -- RthSubstrate1/LConn1 -- Rth_basePlt/RConn1 -- "Hc1 "/RConn1 -- RthSubstrate1/RConn1 -- ThermalModel_BodyDiode_CL/RConn1
  Simulink-PS Converter5/RConn1 -- Controlled Heat Flow Rate Source9/RConn1
  Controlled Heat Flow Rate Source7/RConn1 -- Simulink-PS Converter4/RConn1
  Controlled Heat Flow Rate Source7/RConn2 -- Thermal Reference9/LConn1
  Controlled Heat Flow Rate Source7/LConn1 -- ThermalModel_BodyDiode_CH/LConn1
  Hi1/RConn1 -- Controlled Heat Flow Rate Source8/RConn1

== system MotorDriveThermalTestbench/Motor Cooling/windingOilJet/ThermalResistance /    HeatTransferCoefficient ==
  PS Divide : fl_lib/Physical Signals/Functions/PS Divide
  PS Gain : fl_lib/Physical Signals/Functions/PS Gain  gain=0.126 W/(m*K)
  Nu : PMIOPort  Side=Left
  od : PMIOPort  Port=2  Side=Left
  HTC : PMIOPort  Port=3  Side=Right
  connections:
  PS Divide/LConn1 -- PS Gain/RConn1
  Nu/RConn1 -- PS Gain/LConn1
  PS Divide/RConn1 -- HTC/RConn1
  od/RConn1 -- PS Divide/LConn2

== system MotorDriveThermalTestbench/Motor Cooling/windingOilJet/ThermalResistance /Nusselt No ==
  PS Gain : fl_lib/Physical Signals/Functions/PS Gain  gain=0.683
  PS Math Function : fl_lib/Physical Signals/Functions/PS Math Function  fcn_choice=foundation.enum.math_function.pow  v=0.466
  PS Math Function1 : fl_lib/Physical Signals/Functions/PS Math Function  fcn_choice=foundation.enum.math_function.pow  v=1/3
  PS Product : fl_lib/Physical Signals/Functions/PS Product
  Re : PMIOPort  Side=Left
  Nu : PMIOPort  Port=2  Side=Right
  Pr : PMIOPort  Port=3  Side=Left
  connections:
  PS Product/RConn1 -- Nu/RConn1
  PS Gain/RConn1 -- PS Product/LConn1
  PS Math Function1/RConn1 -- PS Product/LConn2
  Pr/RConn1 -- PS Math Function1/LConn1
  PS Math Function/RConn1 -- PS Gain/LConn1
  Re/RConn1 -- PS Math Function/LConn1
